simulink model "Stabilizator_cisnienia"  (R2016a)
settings: Solver=VariableStepAuto  StartTime=0.0  StopTime=400  RelTol=1e-3
values from neighbouring files (symbols this model uses):
  A_pr = 38.484    [Pressurizer_constants.m]
  AUX0 = 0    [Pressurizer_constants.m]
  AUX_pr0 = 0    [Pressurizer_constants.m]
  B_cl = -0.0631    [Pressurizer_constants.m]    (also in zmienne.m)
  B_hl = -0.0741    [Pressurizer_constants.m]    (also in zmienne.m)
  G_he = -250    [Pressurizer_constants.m]
  G_sp = 0    [Pressurizer_constants.m]
  H_fgp0 = 414.8    [Pressurizer_constants.m]
  H_sp = 574.36    [Pressurizer_constants.m]
  H_wi0 = 672.84    [Pressurizer_constants.m]
  H_wp0 = 701.1    [Pressurizer_constants.m]
  J = 5.4027    [Pressurizer_constants.m]    (also in zmienne.m = 5.404)
  K_p1 = -0.008152    [Pressurizer_constants.m]
  K_p2 = 0.00470802    [Pressurizer_constants.m]
  K_p3 = 0.118    [Pressurizer_constants.m]
  K_p4 = -0.2081    [Pressurizer_constants.m]
  K_p5 = 5.9e-6    (= 5.9e-06)    [Pressurizer_constants.m]
  K_p6 = -1.118e-4    (= -0.0001118)    [Pressurizer_constants.m]
  K_pr = 0    [Pressurizer_constants.m]
  L_p = 46.76    [Pressurizer_constants.m]
  L_sp0 = 18.7    [Pressurizer_constants.m]
  L_wp0 = 28.06    [Pressurizer_constants.m]
  M_sp0 = 4588.33    [Pressurizer_constants.m]
  M_wp0 = 40029.65    [Pressurizer_constants.m]
  Pr0 = 2250    [Pressurizer_constants.m]
  ro_sp0 = 6.37267    [Pressurizer_constants.m]
  ro_wp0 = 37.064    [Pressurizer_constants.m]
  tau1_pr = 900    [Pressurizer_constants.m]
  tau2_pr = 2    [Pressurizer_constants.m]
  tau3_pr = 200    [Pressurizer_constants.m]
  tau4_pr = 2    [Pressurizer_constants.m]
  V_cl = 2000    [Pressurizer_constants.m]    (also in zmienne.m)
  V_fp0 = 0.02698    [Pressurizer_constants.m]
  V_gp0 = 0.15692    [Pressurizer_constants.m]
  V_hl = 1000    [Pressurizer_constants.m]    (also in zmienne.m)
  V_lp = 1791    [Pressurizer_constants.m]    (also in zmienne.m)
  V_mo = 540    [Pressurizer_constants.m]    (also in zmienne.m)
  V_p = 1077    [Pressurizer_constants.m]    (also in zmienne.m)
  V_sp0 = 720    [Pressurizer_constants.m]
  V_up = 1376    [Pressurizer_constants.m]    (also in zmienne.m)
  V_wp0 = 1080    [Pressurizer_constants.m]
  W_sr0 = 0    [Pressurizer_constants.m]
  X_fgp = 883.025    [Pressurizer_constants.m]
  X_fp = 435.6    [Pressurizer_constants.m]
  X_sp = -4.2203    [Pressurizer_constants.m]
  X_vfp = 0.013705    [Pressurizer_constants.m]
  X_vgp = 0.40847    [Pressurizer_constants.m]
  X_wp = 55.406    [Pressurizer_constants.m]
settings Model: Creator=Michal Chruscinski  LastModifiedBy=Michal Chruscinski

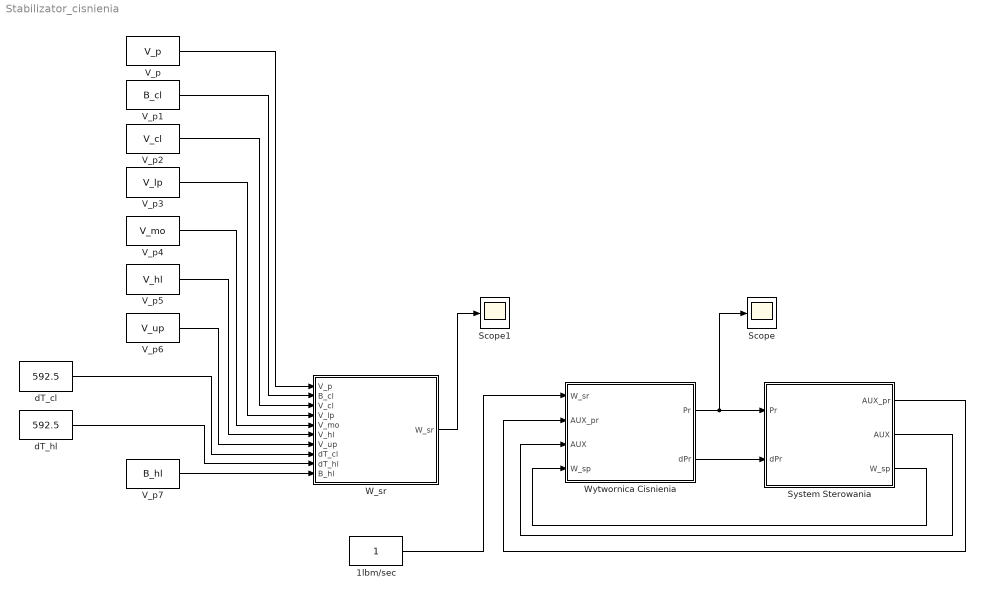
== system Stabilizator_cisnienia ==
  1lbm/sec : Constant
  Scope : Scope
  Scope1 : Scope
  System Sterowania : Subsystem
  V_p : Constant  Value=V_p
  V_p1 : Constant  Value=B_cl
  V_p2 : Constant  Value=V_cl
  V_p3 : Constant  Value=V_lp
  V_p4 : Constant  Value=V_mo
  V_p5 : Constant  Value=V_hl
  V_p6 : Constant  Value=V_up
  V_p7 : Constant  Value=B_hl
  W_sr : Subsystem
  Wytwornica Cisnienia : Subsystem
  dT_cl : Constant  Value=592.5
  dT_hl : Constant  Value=592.5
  wires:
  V_p/1 -> W_sr/1(V_p)
  V_p1/1 -> W_sr/2(B_cl)
  V_p2/1 -> W_sr/3(V_cl)
  V_p3/1 -> W_sr/4(V_lp)
  V_p4/1 -> W_sr/5(V_mo)
  V_p5/1 -> W_sr/6(V_hl)
  V_p6/1 -> W_sr/7(V_up)
  dT_cl/1 -> W_sr/8(dT_cl)
  dT_hl/1 -> W_sr/9(dT_hl)
  V_p7/1 -> W_sr/10(B_hl)
  Wytwornica Cisnienia/1(Pr) -> Scope/1, System Sterowania/1(Pr)
  Wytwornica Cisnienia/2(dPr) -> System Sterowania/2(dPr)
  W_sr/1(W_sr) -> Scope1/1
  System Sterowania/1(AUX_pr) -> Wytwornica Cisnienia/2(AUX_pr)
  System Sterowania/2(AUX) -> Wytwornica Cisnienia/3(AUX)
  System Sterowania/3(W_sp) -> Wytwornica Cisnienia/4(W_sp)
  1lbm/sec/1 -> Wytwornica Cisnienia/1(W_sr)

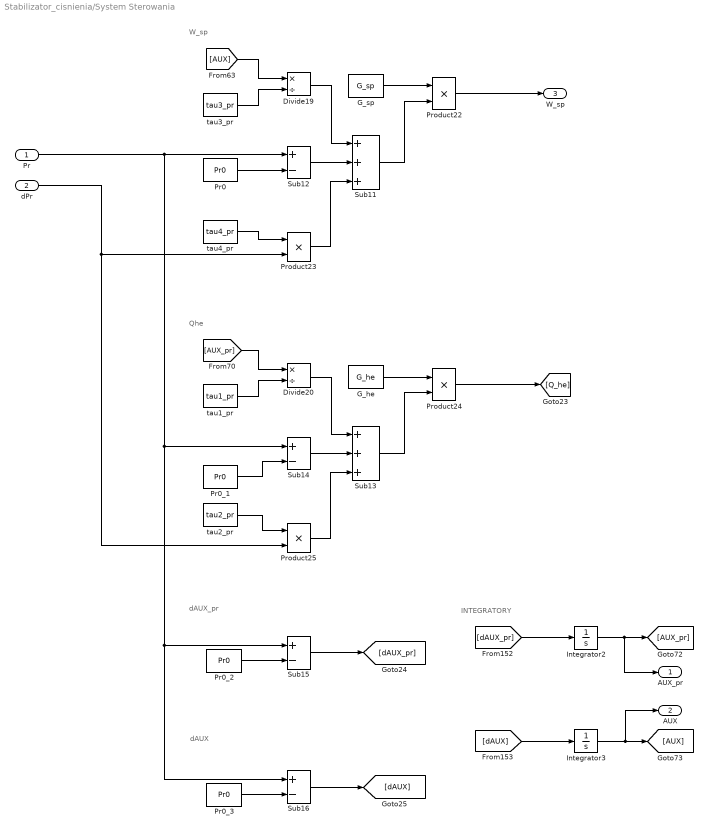
== system Stabilizator_cisnienia/System Sterowania ==
  note: INTEGRATORY
  note: dAUX
  note: dAUX_pr
  note: W_sp
  note: Qhe
  Pr : Inport
  dPr : Inport  Port=2
  Divide19 : Product  Inputs=*/
  Divide20 : Product  Inputs=*/
  G_he : Constant  Value=G_he
  G_sp : Constant  Value=G_sp
  Integrator2 : Integrator  InitialCondition=AUX_pr0
  Integrator3 : Integrator  InitialCondition=AUX0
  Pr0 : Constant  Value=Pr0
  Pr0_1 : Constant  Value=Pr0
  Pr0_2 : Constant  Value=Pr0
  Pr0_3 : Constant  Value=Pr0
  Product{22..25} (4 alike) : Product
  Sub11 : Sum  Inputs=+++
  Sub{12,14..16} (4 alike) : Sum  Inputs=+-
  Sub13 : Sum  Inputs=+++
  tau1_pr : Constant  Value=tau1_pr
  tau2_pr : Constant  Value=tau2_pr
  tau3_pr : Constant  Value=tau3_pr
  tau4_pr : Constant  Value=tau4_pr
  AUX_pr : Outport
  AUX : Outport  Port=2
  W_sp : Outport  Port=3
  wires:
  [AUX] -> Divide19/1
  tau3_pr/1 -> Divide19/2
  Sub14/1 -> Sub13/2
  Sub13/1 -> Product24/2
  Divide19/1 -> Sub11/1
  Product25/1 -> Sub13/3
  tau2_pr/1 -> Product25/1
  Product24/1 -> [Q_he]
  Pr0_2/1 -> Sub15/2
  [AUX_pr] -> Divide20/1
  Pr0_1/1 -> Sub14/2
  Pr/1 -> Sub14/1, Sub16/1, Sub15/1, Sub12/1
  Pr0_3/1 -> Sub16/2
  Product23/1 -> Sub11/3
  tau4_pr/1 -> Product23/1
  Sub11/1 -> Product22/2
  Divide20/1 -> Sub13/1
  tau1_pr/1 -> Divide20/2
  dPr/1 -> Product25/2, Product23/2
  G_sp/1 -> Product22/1
  Pr0/1 -> Sub12/2
  Product22/1 -> W_sp/1
  Sub12/1 -> Sub11/2
  G_he/1 -> Product24/1
  Sub15/1 -> [dAUX_pr]
  Sub16/1 -> [dAUX]
  Integrator2/1 -> AUX_pr/1, [AUX_pr]
  [dAUX_pr] -> Integrator2/1
  [dAUX] -> Integrator3/1
  Integrator3/1 -> AUX/1, [AUX]

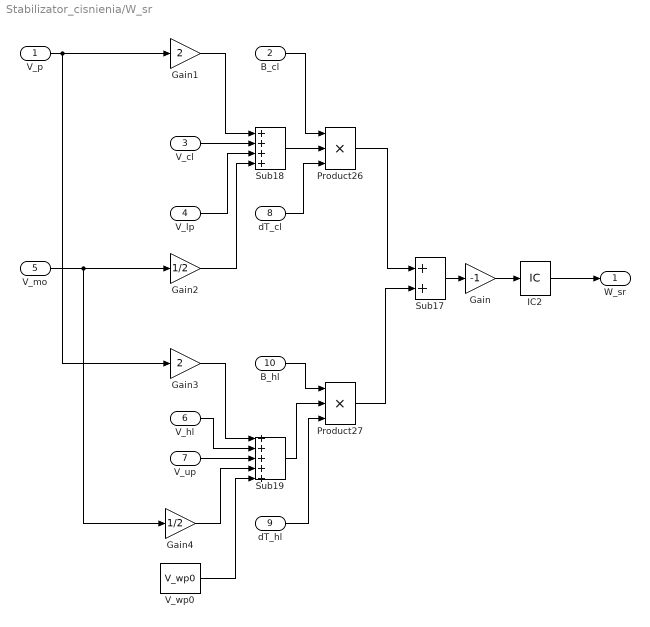
== system Stabilizator_cisnienia/W_sr ==
  V_p : Inport
  B_cl : Inport  Port=2
  V_cl : Inport  Port=3
  V_lp : Inport  Port=4
  V_mo : Inport  Port=5
  V_hl : Inport  Port=6
  V_up : Inport  Port=7
  dT_cl : Inport  Port=8
  dT_hl : Inport  Port=9
  B_hl : Inport  Port=10
  Gain : Gain  Gain=-1
  Gain1 : Gain  Gain=2
  Gain2 : Gain  Gain=1/2
  Gain3 : Gain  Gain=2
  Gain4 : Gain  Gain=1/2
  IC2 : InitialCondition  Value=W_sr0
  Product26 : Product  Inputs=3
  Product27 : Product  Inputs=3
  Sub17 : Sum
  Sub18 : Sum  Inputs=++++
  Sub19 : Sum  Inputs=+++++
  V_wp0 : Constant  Value=V_wp0
  W_sr : Outport
  wires:
  Sub17/1 -> Gain/1
  Gain1/1 -> Sub18/1
  Sub18/1 -> Product26/2
  Product26/1 -> Sub17/1
  Gain/1 -> IC2/1
  Product27/1 -> Sub17/2
  Sub19/1 -> Product27/2
  Gain4/1 -> Sub19/4
  Gain2/1 -> Sub18/4
  Gain3/1 -> Sub19/1
  IC2/1 -> W_sr/1
  V_p/1 -> Gain3/1, Gain1/1
  B_cl/1 -> Product26/1
  V_cl/1 -> Sub18/2
  V_lp/1 -> Sub18/3
  V_mo/1 -> Gain4/1, Gain2/1
  V_hl/1 -> Sub19/2
  V_up/1 -> Sub19/3
  V_wp0/1 -> Sub19/5
  dT_cl/1 -> Product26/3
  dT_hl/1 -> Product27/3
  B_hl/1 -> Product27/1

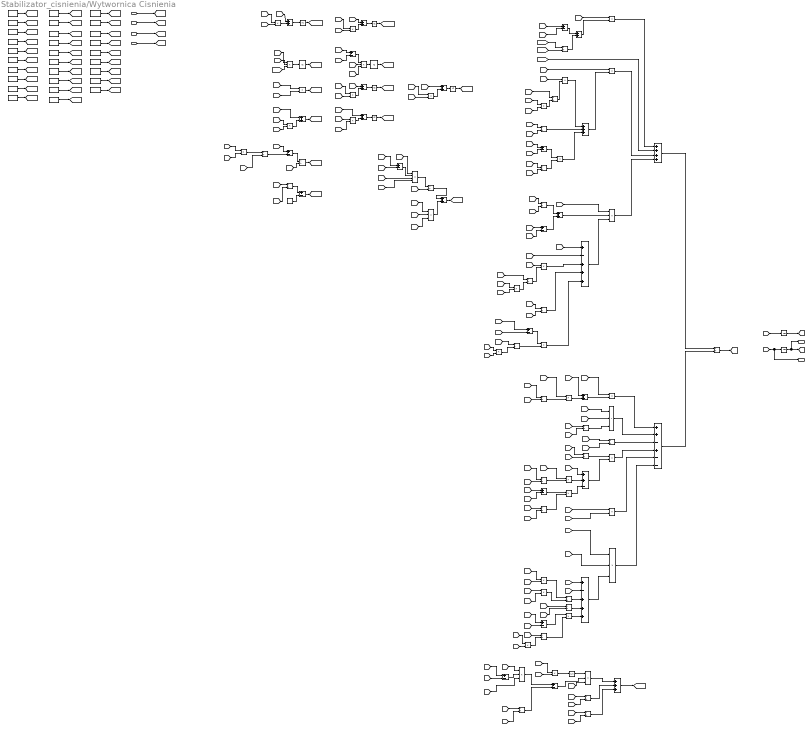
== system Stabilizator_cisnienia/Wytwornica Cisnienia ==
  note: INTEGRATION
  note: dL_wp
  note: EQUATIONS
  note: CONSTANTS
  note: dPr
  note: dPr_mianownik
  note: dPr_licznik
  W_sr : Inport
  AUX_pr : Inport  Port=2
  AUX : Inport  Port=3
  W_sp : Inport  Port=4
  A_pr : Constant  Value=A_pr
  Add1 : Sum
  Add2 : Sum  Inputs=++++
  Add3 : Sum  Inputs=+++
  Add4 : Sum
  Add5 : Sum
  Apr*(Lp-Lwp)*Kp2 : Product  Inputs=3
  Apr*(Lp-Lwp)*Kp2*ROUwp/ROUsp1 : Product  Inputs=*/
  Apr*(Lp-Lwp)*Kp2*ROUwp1 : Product  Inputs=4
  Apr*Lwp*Kp2 : Product  Inputs=3
  C1p : Sum  Inputs=+-
  C2p/C1p : Product  Inputs=*/
  C2p1 : Sum
  DLwp : Sum  Inputs=+++
  DLwp_drugi_nawias : Sum  Inputs=+-
  DLwp_glowny_iloczyn : Product  Inputs=3
  Divide{1..18} (18 alike) : Product  Inputs=*/
  G_he : Constant  Value=G_he
  "G_sp " : Constant  Value=G_sp
  H_fsr : Sum
  H_sp : Constant  Value=H_sp
  H_wi0 : Constant  Value=H_wi0
  H_wp0 : Constant  Value=H_wp0
  Hfsr : Sum
  IC : InitialCondition  Value=M_wp0
  IC1 : InitialCondition  Value=M_sp0
  IC3 : InitialCondition  Value=V_gp0
  IC4 : InitialCondition  Value=V_fp0
  IC5 : InitialCondition  Value=ro_sp0
  IC6 : InitialCondition  Value=ro_wp0
  IC7 : InitialCondition  Value=H_fgp0
  Integrator : Integrator  InitialCondition=L_wp0
  Integrator1 : Integrator  InitialCondition=Pr0
  J : Constant  Value=J
  K_p1 : Constant  Value=K_p1
  K_p2 : Constant  Value=K_p2
  K_p3 : Constant  Value=K_p3
  K_p4 : Constant  Value=K_p4
  K_p5 : Constant  Value=K_p5
  K_p6 : Constant  Value=K_p6
  K_pr : Constant  Value=K_pr
  Kp1 - ROUwp*Kp2/ROUsp : Sum  Inputs=+-
  Kp1*Pr : Product
  Kp2*Pr : Product
  Kp3 * Pr : Product
  Kp4 * Pr : Product
  Kp5 * Pr : Product
  Kp5 * Pr2 : Product
  Kp7 : Product  Inputs=*/
  L_p : Constant  Value=L_p
  L_sp0 : Constant  Value=L_sp0
  Liczba_1 : Constant
  Lp-Lwp : Sum  Inputs=+-
  Lp-Lwp1 : Sum  Inputs=+-
  Lp-Lwp2 : Sum  Inputs=+-
  Math Function : Math  Operator=reciprocal  SaturateOnIntegerOverflow=on
  Msp : Product  Inputs=3
  Mwp : Product  Inputs=3
  Pr0 : Constant  Value=Pr0
  Product{,1..5,7..11,13..16,18..21} (19 alike) : Product
  Product12 : Product  Inputs=3
  Product17 : Product  Inputs=3
  Product6 : Product  Inputs=3
  ROUsp : Sum
  ROUsp*Apr : Product
  ROUwp : Sum
  ROUwp*Kp2 : Product
  ROUwp*Kp2/ROUsp : Product  Inputs=*/
  ROUwp/ROUsp : Product  Inputs=*/
  Sub{1..3,5,8,10} (6 alike) : Sum  Inputs=+-
  Sub4 : Sum  Inputs=+-+++
  Sub6 : Sum  Inputs=++-+--
  Sub7 : Sum  Inputs=++-
  Sub9 : Sum  Inputs=+-+++
  V_sp0 : Constant  Value=V_sp0
  V_wp0 : Constant  Value=V_wp0
  Vfp : Sum
  Vfp1 : Sum
  Vwp : Product
  Wsp/C1p : Product  Inputs=*/
  Wsr/C1p1 : Product  Inputs=*/
  X_fgp : Constant  Value=X_fgp
  X_fp : Constant  Value=X_fp
  X_sp : Constant  Value=X_sp
  X_vfp : Constant  Value=X_vfp
  X_vgp : Constant  Value=X_vgp
  X_wp : Constant  Value=X_wp
  tau1_pr : Constant  Value=tau1_pr
  tau2_pr : Constant  Value=tau2_pr
  tau3_pr : Constant  Value=tau3_pr
  tau4_pr : Constant  Value=tau4_pr
  Pr : Outport
  dPr : Outport  Port=2
  wires:
  K_pr/1 -> [K_pr]
  G_he/1 -> [G_he]
  IC7/1 -> [H_fgp]
  IC5/1 -> [ro_sp]
  ROUsp/1 -> IC5/1
  IC3/1 -> [V_gp]
  IC6/1 -> [ro_wp]
  IC/1 -> [M_wp]
  C1p/1 -> [C1_p]
  Wsr/C1p1/1 -> DLwp/2
  [X_vfp] -> Vfp/1
  [K_p2] -> Kp2*Pr/1
  [K_p3] -> Kp3 * Pr/1
  Liczba_1/1 -> C1p/2
  Kp2*Pr/1 -> ROUsp/2
  ROUwp*Kp2/1 -> ROUwp*Kp2/ROUsp/1
  Kp5 * Pr/1 -> Vfp/2
  ROUwp*Kp2/ROUsp/1 -> Kp1 - ROUwp*Kp2/ROUsp/2
  [X_fp] -> H_fsr/1
  Apr*(Lp-Lwp)*Kp2/1 -> DLwp_drugi_nawias/1
  C2p/C1p/1 -> DLwp_drugi_nawias/2
  Kp3 * Pr/1 -> H_fsr/2
  DLwp_drugi_nawias/1 -> DLwp_glowny_iloczyn/2
  Divide9/1 -> [dPr]
  Kp1*Pr/1 -> ROUwp/2
  [K_p1] -> Kp1*Pr/1
  Kp4 * Pr/1 -> Hfsr/2
  DLwp_glowny_iloczyn/1 -> DLwp/1
  [K_p4] -> Kp4 * Pr/1
  Wsp/C1p/1 -> DLwp/3
  ROUwp/1 -> IC6/1
  ROUwp/ROUsp/1 -> C1p/1
  ROUsp*Apr/1 -> Math Function/1
  DLwp/1 -> [dL_wp]
  Math Function/1 -> DLwp_glowny_iloczyn/1
  [X_sp] -> ROUsp/1
  [W_sp] -> Wsp/C1p/1
  [X_fgp] -> Hfsr/1
  Kp1 - ROUwp*Kp2/ROUsp/1 -> Kp7/1
  [C1_p] -> Divide3/2
  [V_fp] -> Sub2/2
  Vwp/1 -> [V_wp]
  Add1/1 -> Product/2
  [tau1_pr] -> Divide2/2
  [Pr] -> Divide4/1
  [C1_p] -> Divide4/2
  Hfsr/1 -> IC7/1
  Msp/1 -> IC1/1
  [K_pr] -> Add2/2
  Product3/1 -> Divide1/2
  [Pr] -> Product2/1
  Divide2/1 -> Add1/2
  Product2/1 -> Add3/1
  [V_fp] -> Divide1/1
  [H_fgp] -> Divide3/1
  Sub1/1 -> Add1/1
  Mwp/1 -> IC/1
  H_fsr/1 -> [H_fsr]
  [Pr] -> Sub1/1
  Product/1 -> Add2/1
  Vfp/1 -> IC4/1
  Kp7/1 -> [K_p7]
  [C1_p] -> Product3/1
  [W_sr] -> Product1/1
  [AUX_pr] -> Divide2/1
  Divide3/1 -> Add3/2
  Divide4/1 -> Product4/2
  [V_gp] -> Sub2/1
  Sub2/1 -> Product4/1
  [Pr0] -> Sub1/2
  Divide1/1 -> Product2/2
  Sub4/1 -> Product6/3
  Sub5/1 -> Product9/1
  [Pr] -> Divide8/1
  [V_gp] -> Divide6/1
  [V_gp] -> Sub5/1
  [V_fp] -> Sub5/2
  [Pr] -> Product7/1
  [J] -> Product3/2
  Product10/1 -> Divide8/2
  Product7/1 -> Sub4/3
  [H_fsr] -> Sub4/2
  [H_fgp] -> Divide7/1
  Product1/1 -> Add2/3
  [tau3_pr] -> Divide5/2
  Product8/1 -> Divide6/2
  [C1_p] -> Product8/1
  [J] -> Product8/2
  [C1_p] -> Product10/1
  Divide7/1 -> Sub4/4
  [AUX] -> Divide5/1
  Add4/1 -> Product6/2
  Divide5/1 -> Add4/1
  Add3/1 -> Product1/2
  [C1_p] -> Divide7/2
  Sub3/1 -> Add4/2
  Divide6/1 -> Product7/2
  Product4/1 -> Add3/3
  [Pr0] -> Sub3/2
  [Pr] -> Sub3/1
  [J] -> Product10/2
  Product9/1 -> Sub4/5
  Divide8/1 -> Product9/2
  Sub8/1 -> Product15/1
  Product5/1 -> Sub6/1
  Divide10/1 -> Product11/2
  [Pr] -> Divide10/1
  [C1_p] -> Divide13/1
  [V_fp] -> Divide14/1
  [Pr] -> Product14/1
  Add5/1 -> Product5/2
  [J] -> Divide11/2
  Divide12/1 -> Sub6/3
  [V_wp] -> Divide12/1
  Product11/1 -> Add5/2
  [Pr] -> Divide11/1
  [M_sp] -> Product12/1
  Product14/1 -> Sub7/2
  Add2/1 -> Divide9/1
  Sub6/1 -> Divide9/2
  [J] -> Divide12/2
  Sub7/1 -> Product13/2
  Product12/1 -> Sub6/2
  [M_wp] -> Product5/1
  [H_fgp] -> Sub7/1
  Product6/1 -> Add2/4
  [J] -> Divide10/2
  Divide13/1 -> Product13/1
  Divide11/1 -> Product12/3
  [C2_p] -> Divide13/2
  Product13/1 -> Sub6/4
  Divide14/1 -> Product14/2
  [J] -> Divide14/2
  [K_p6] -> Product12/2
  Product15/1 -> Sub7/3
  [G_sp] -> Product17/1
  [tau2_pr] -> Product16/2
  Divide16/1 -> Sub9/3
  Sub10/1 -> Product20/1
  Product21/1 -> Divide18/2
  Sub9/1 -> Product17/3
  [V_gp] -> Sub10/1
  [J] -> Product18/2
  [J] -> Divide15/2
  [H_sp] -> Sub4/1
  Product18/1 -> Divide16/2
  [Pr] -> Divide15/1
  [G_he] -> Product/1
  Product16/1 -> Sub6/5
  [H_fsr] -> Sub9/2
  [Pr] -> Product19/1
  [G_he] -> Product16/1
  Divide15/1 -> Product15/2
  Product17/1 -> Sub6/6
  [G_sp] -> Product6/1
  [H_fgp] -> Divide17/1
  [V_fp] -> Sub8/1
  [C1_p] -> Product18/1
  [C1_p] -> Divide17/2
  Product19/1 -> Divide16/1
  [V_gp] -> Product19/2
  [tau4_pr] -> Product17/2
  [H_sp] -> Sub9/1
  Divide17/1 -> Sub9/4
  Product20/1 -> Sub9/5
  [V_gp] -> Sub8/2
  Divide18/1 -> Product20/2
  [J] -> Product21/2
  [C1_p] -> Product21/1
  [V_fp] -> Sub10/2
  [Pr] -> Kp1*Pr/2
  L_sp0/1 -> [L_sp0]
  H_wp0/1 -> [H_wp0]
  A_pr/1 -> [A_pr]
  V_sp0/1 -> [V_sp0]
  V_wp0/1 -> [V_wp0]
  K_p4/1 -> [K_p4]
  K_p6/1 -> [K_p6]
  X_sp/1 -> [X_sp]
  X_vfp/1 -> [X_vfp]
  Pr0/1 -> [Pr0]
  K_p5/1 -> [K_p5]
  L_p/1 -> [L_p]
  X_fp/1 -> [X_fp]
  X_vgp/1 -> [X_vgp]
  J/1 -> [J]
  X_wp/1 -> [X_wp]
  tau1_pr/1 -> [tau1_pr]
  tau2_pr/1 -> [tau2_pr]
  tau3_pr/1 -> [tau3_pr]
  [Pr] -> Kp2*Pr/2
  [X_wp] -> ROUwp/1
  X_fgp/1 -> [X_fgp]
  [X_vgp] -> Vfp1/1
  Apr*Lwp*Kp2/1 -> C2p1/2
  C2p1/1 -> [C2_p]
  [ro_wp] -> ROUwp/ROUsp/1
  [K_p1] -> Apr*Lwp*Kp2/3
  [A_pr] -> Apr*Lwp*Kp2/1
  [Pr] -> Kp4 * Pr/2
  [L_p] -> Lp-Lwp/1
  [A_pr] -> Msp/2
  [K_p5] -> Kp5 * Pr/1
  [Pr] -> Kp5 * Pr/2
  Vfp1/1 -> IC3/1
  [L_wp] -> Mwp/1
  Lp-Lwp/1 -> Msp/1
  [K_p1] -> Kp1 - ROUwp*Kp2/ROUsp/1
  [ro_wp] -> ROUwp*Kp2/1
  Kp5 * Pr2/1 -> Vfp1/2
  [L_wp] -> Lp-Lwp/2
  [ro_sp] -> Kp7/2
  [A_pr] -> Vwp/2
  [ro_wp] -> Mwp/3
  [Pr] -> Kp3 * Pr/2
  [K_p6] -> Kp5 * Pr2/1
  [Pr] -> Kp5 * Pr2/2
  [ro_sp] -> ROUwp*Kp2/ROUsp/2
  [ro_sp] -> ROUwp/ROUsp/2
  [A_pr] -> Mwp/2
  [ro_sp] -> Msp/3
  [K_p2] -> ROUwp*Kp2/2
  [L_wp] -> Vwp/1
  Apr*(Lp-Lwp)*Kp2*ROUwp1/1 -> Apr*(Lp-Lwp)*Kp2*ROUwp/ROUsp1/1
  Apr*(Lp-Lwp)*Kp2*ROUwp/ROUsp1/1 -> C2p1/1
  [L_wp] -> Lp-Lwp1/2
  [L_wp] -> Lp-Lwp2/2
  [W_sr] -> Wsr/C1p1/1
  [K_p2] -> Apr*(Lp-Lwp)*Kp2/3
  [ro_sp] -> Apr*(Lp-Lwp)*Kp2*ROUwp/ROUsp1/2
  Lp-Lwp2/1 -> Apr*(Lp-Lwp)*Kp2/2
  [K_p2] -> Apr*(Lp-Lwp)*Kp2*ROUwp1/3
  [A_pr] -> Apr*(Lp-Lwp)*Kp2*ROUwp1/1
  [L_p] -> Lp-Lwp2/1
  Lp-Lwp1/1 -> Apr*(Lp-Lwp)*Kp2*ROUwp1/2
  [ro_wp] -> Apr*(Lp-Lwp)*Kp2*ROUwp1/4
  [C1_p] -> Wsp/C1p/2
  [dPr] -> DLwp_glowny_iloczyn/3
  [C1_p] -> C2p/C1p/2
  [L_p] -> Lp-Lwp1/1
  [ro_sp] -> ROUsp*Apr/2
  [L_wp] -> Apr*Lwp*Kp2/2
  [C2_p] -> C2p/C1p/1
  [C1_p] -> Wsr/C1p1/2
  [A_pr] -> ROUsp*Apr/1
  [A_pr] -> Apr*(Lp-Lwp)*Kp2/1
  H_wi0/1 -> [H_wi0]
  H_sp/1 -> [H_sp]
  [dL_wp] -> Integrator/1
  Integrator/1 -> [L_wp]
  K_p3/1 -> [K_p3]
  K_p2/1 -> [K_p2]
  [K_p3] -> Add5/1
  [dPr] -> dPr/1, Integrator1/1
  K_p1/1 -> [K_p1]
  [K_p5] -> Product11/1
  Integrator1/1 -> Pr/1, [Pr]
  tau4_pr/1 -> [tau4_pr]
  [Pr] -> Divide18/1
  IC1/1 -> [M_sp]
  IC4/1 -> [V_fp]
  "G_sp "/1 -> [G_sp]
  W_sr/1 -> [W_sr]
  AUX/1 -> [AUX]
  AUX_pr/1 -> [AUX_pr]
  W_sp/1 -> [W_sp]
